simulink model "gm_parallel_8_phase_voltages"  (R2022a)
settings: Solver=FixedStepDiscrete  StartTime=0.0  StopTime=10.0  RelTol=1e-3
undefined symbols (not defined in the file or in its folder): f_c, u_dc
libraries: hdlmdlgenlib x14, simulink x2
(part 4 of 4)

== system gm_parallel_8_phase_voltages/Phase_voltages_per_switching_state1/Subsystem/MATLAB Function10/adder1 ==
  In1 : Inport
  In2 : Inport  Port=2
  adder1 : Sum  OutDataTypeStr=single  SampleTime=1e-08
  adder1_pd1 : Delay  DelayLength=6
  Out1 : Outport
  wires:
  In1/1 -> adder1/1
  In2/1 -> adder1/2
  adder1/1 -> adder1_pd1/1
  adder1_pd1/1 -> Out1/1

== system gm_parallel_8_phase_voltages/Phase_voltages_per_switching_state1/Subsystem/MATLAB Function10/adder2 ==
  In1 : Inport
  In2 : Inport  Port=2
  adder2 : Sum  OutDataTypeStr=single  SampleTime=1e-08
  adder2_pd1 : Delay  DelayLength=6
  Out1 : Outport
  wires:
  In1/1 -> adder2/1
  In2/1 -> adder2/2
  adder2/1 -> adder2_pd1/1
  adder2_pd1/1 -> Out1/1

== system gm_parallel_8_phase_voltages/Phase_voltages_per_switching_state1/Subsystem/MATLAB Function10/multiplier ==
  In1 : Inport
  In2 : Inport  Port=2
  multiplier : Product  Inputs=**  OutDataTypeStr=single  SampleTime=1e-08
  multiplier_pd1 : Delay  DelayLength=6
  Out1 : Outport
  wires:
  In1/1 -> multiplier/1
  In2/1 -> multiplier/2
  multiplier/1 -> multiplier_pd1/1
  multiplier_pd1/1 -> Out1/1

== system gm_parallel_8_phase_voltages/Phase_voltages_per_switching_state1/Subsystem/MATLAB Function10/multiplier1 ==
  In1 : Inport
  In2 : Inport  Port=2
  multiplier1 : Product  Inputs=**  OutDataTypeStr=single  SampleTime=1e-08
  multiplier1_pd1 : Delay  DelayLength=6
  Out1 : Outport
  wires:
  In1/1 -> multiplier1/1
  In2/1 -> multiplier1/2
  multiplier1/1 -> multiplier1_pd1/1
  multiplier1_pd1/1 -> Out1/1

== system gm_parallel_8_phase_voltages/Phase_voltages_per_switching_state1/Subsystem/MATLAB Function10/multiplier2 ==
  In1 : Inport
  In2 : Inport  Port=2
  multiplier2 : Product  Inputs=**  OutDataTypeStr=single  SampleTime=1e-08
  multiplier2_pd1 : Delay  DelayLength=6
  Out1 : Outport
  wires:
  In1/1 -> multiplier2/1
  In2/1 -> multiplier2/2
  multiplier2/1 -> multiplier2_pd1/1
  multiplier2_pd1/1 -> Out1/1

== system gm_parallel_8_phase_voltages/Phase_voltages_per_switching_state1/Subsystem/MATLAB Function10/multiplier3 ==
  In1 : Inport
  In2 : Inport  Port=2
  multiplier3 : Product  Inputs=**  OutDataTypeStr=single  SampleTime=1e-08
  multiplier3_pd1 : Delay  DelayLength=6
  Out1 : Outport
  wires:
  In1/1 -> multiplier3/1
  In2/1 -> multiplier3/2
  multiplier3/1 -> multiplier3_pd1/1
  multiplier3_pd1/1 -> Out1/1

== system gm_parallel_8_phase_voltages/Phase_voltages_per_switching_state1/Subsystem/MATLAB Function10/multiplier4 ==
  In1 : Inport
  In2 : Inport  Port=2
  multiplier4 : Product  Inputs=**  OutDataTypeStr=single  SampleTime=1e-08
  multiplier4_pd1 : Delay  DelayLength=6
  Out1 : Outport
  wires:
  In1/1 -> multiplier4/1
  In2/1 -> multiplier4/2
  multiplier4/1 -> multiplier4_pd1/1
  multiplier4_pd1/1 -> Out1/1

== system gm_parallel_8_phase_voltages/Phase_voltages_per_switching_state1/Subsystem/MATLAB Function10/uminus ==
  In1 : Inport
  uminus : UnaryMinus  SampleTime=1e-08
  Out1 : Outport
  wires:
  In1/1 -> uminus/1
  uminus/1 -> Out1/1

== system gm_parallel_8_phase_voltages/Phase_voltages_per_switching_state1/Subsystem/MATLAB Function11/adder1 ==
  In1 : Inport
  In2 : Inport  Port=2
  adder1 : Sum  OutDataTypeStr=single  SampleTime=1e-08
  adder1_pd1 : Delay  DelayLength=6
  Out1 : Outport
  wires:
  In1/1 -> adder1/1
  In2/1 -> adder1/2
  adder1/1 -> adder1_pd1/1
  adder1_pd1/1 -> Out1/1

== system gm_parallel_8_phase_voltages/Phase_voltages_per_switching_state1/Subsystem/MATLAB Function11/adder2 ==
  In1 : Inport
  In2 : Inport  Port=2
  adder2 : Sum  OutDataTypeStr=single  SampleTime=1e-08
  adder2_pd1 : Delay  DelayLength=6
  Out1 : Outport
  wires:
  In1/1 -> adder2/1
  In2/1 -> adder2/2
  adder2/1 -> adder2_pd1/1
  adder2_pd1/1 -> Out1/1

== system gm_parallel_8_phase_voltages/Phase_voltages_per_switching_state1/Subsystem/MATLAB Function11/multiplier ==
  In1 : Inport
  In2 : Inport  Port=2
  multiplier : Product  Inputs=**  OutDataTypeStr=single  SampleTime=1e-08
  multiplier_pd1 : Delay  DelayLength=6
  Out1 : Outport
  wires:
  In1/1 -> multiplier/1
  In2/1 -> multiplier/2
  multiplier/1 -> multiplier_pd1/1
  multiplier_pd1/1 -> Out1/1

== system gm_parallel_8_phase_voltages/Phase_voltages_per_switching_state1/Subsystem/MATLAB Function11/multiplier1 ==
  In1 : Inport
  In2 : Inport  Port=2
  multiplier1 : Product  Inputs=**  OutDataTypeStr=single  SampleTime=1e-08
  multiplier1_pd1 : Delay  DelayLength=6
  Out1 : Outport
  wires:
  In1/1 -> multiplier1/1
  In2/1 -> multiplier1/2
  multiplier1/1 -> multiplier1_pd1/1
  multiplier1_pd1/1 -> Out1/1

== system gm_parallel_8_phase_voltages/Phase_voltages_per_switching_state1/Subsystem/MATLAB Function11/multiplier2 ==
  In1 : Inport
  In2 : Inport  Port=2
  multiplier2 : Product  Inputs=**  OutDataTypeStr=single  SampleTime=1e-08
  multiplier2_pd1 : Delay  DelayLength=6
  Out1 : Outport
  wires:
  In1/1 -> multiplier2/1
  In2/1 -> multiplier2/2
  multiplier2/1 -> multiplier2_pd1/1
  multiplier2_pd1/1 -> Out1/1

== system gm_parallel_8_phase_voltages/Phase_voltages_per_switching_state1/Subsystem/MATLAB Function11/multiplier3 ==
  In1 : Inport
  In2 : Inport  Port=2
  multiplier3 : Product  Inputs=**  OutDataTypeStr=single  SampleTime=1e-08
  multiplier3_pd1 : Delay  DelayLength=6
  Out1 : Outport
  wires:
  In1/1 -> multiplier3/1
  In2/1 -> multiplier3/2
  multiplier3/1 -> multiplier3_pd1/1
  multiplier3_pd1/1 -> Out1/1

== system gm_parallel_8_phase_voltages/Phase_voltages_per_switching_state1/Subsystem/MATLAB Function11/multiplier4 ==
  In1 : Inport
  In2 : Inport  Port=2
  multiplier4 : Product  Inputs=**  OutDataTypeStr=single  SampleTime=1e-08
  multiplier4_pd1 : Delay  DelayLength=6
  Out1 : Outport
  wires:
  In1/1 -> multiplier4/1
  In2/1 -> multiplier4/2
  multiplier4/1 -> multiplier4_pd1/1
  multiplier4_pd1/1 -> Out1/1

== system gm_parallel_8_phase_voltages/Phase_voltages_per_switching_state1/Subsystem/MATLAB Function11/uminus ==
  In1 : Inport
  uminus : UnaryMinus  SampleTime=1e-08
  Out1 : Outport
  wires:
  In1/1 -> uminus/1
  uminus/1 -> Out1/1

== system gm_parallel_8_phase_voltages/Phase_voltages_per_switching_state1/Subsystem/MATLAB Function12/adder1 ==
  In1 : Inport
  In2 : Inport  Port=2
  adder1 : Sum  OutDataTypeStr=single  SampleTime=1e-08
  adder1_pd1 : Delay  DelayLength=6
  Out1 : Outport
  wires:
  In1/1 -> adder1/1
  In2/1 -> adder1/2
  adder1/1 -> adder1_pd1/1
  adder1_pd1/1 -> Out1/1

== system gm_parallel_8_phase_voltages/Phase_voltages_per_switching_state1/Subsystem/MATLAB Function12/adder2 ==
  In1 : Inport
  In2 : Inport  Port=2
  adder2 : Sum  OutDataTypeStr=single  SampleTime=1e-08
  adder2_pd1 : Delay  DelayLength=6
  Out1 : Outport
  wires:
  In1/1 -> adder2/1
  In2/1 -> adder2/2
  adder2/1 -> adder2_pd1/1
  adder2_pd1/1 -> Out1/1

== system gm_parallel_8_phase_voltages/Phase_voltages_per_switching_state1/Subsystem/MATLAB Function12/multiplier ==
  In1 : Inport
  In2 : Inport  Port=2
  multiplier : Product  Inputs=**  OutDataTypeStr=single  SampleTime=1e-08
  multiplier_pd1 : Delay  DelayLength=6
  Out1 : Outport
  wires:
  In1/1 -> multiplier/1
  In2/1 -> multiplier/2
  multiplier/1 -> multiplier_pd1/1
  multiplier_pd1/1 -> Out1/1

== system gm_parallel_8_phase_voltages/Phase_voltages_per_switching_state1/Subsystem/MATLAB Function12/multiplier1 ==
  In1 : Inport
  In2 : Inport  Port=2
  multiplier1 : Product  Inputs=**  OutDataTypeStr=single  SampleTime=1e-08
  multiplier1_pd1 : Delay  DelayLength=6
  Out1 : Outport
  wires:
  In1/1 -> multiplier1/1
  In2/1 -> multiplier1/2
  multiplier1/1 -> multiplier1_pd1/1
  multiplier1_pd1/1 -> Out1/1

== system gm_parallel_8_phase_voltages/Phase_voltages_per_switching_state1/Subsystem/MATLAB Function12/multiplier2 ==
  In1 : Inport
  In2 : Inport  Port=2
  multiplier2 : Product  Inputs=**  OutDataTypeStr=single  SampleTime=1e-08
  multiplier2_pd1 : Delay  DelayLength=6
  Out1 : Outport
  wires:
  In1/1 -> multiplier2/1
  In2/1 -> multiplier2/2
  multiplier2/1 -> multiplier2_pd1/1
  multiplier2_pd1/1 -> Out1/1

== system gm_parallel_8_phase_voltages/Phase_voltages_per_switching_state1/Subsystem/MATLAB Function12/multiplier3 ==
  In1 : Inport
  In2 : Inport  Port=2
  multiplier3 : Product  Inputs=**  OutDataTypeStr=single  SampleTime=1e-08
  multiplier3_pd1 : Delay  DelayLength=6
  Out1 : Outport
  wires:
  In1/1 -> multiplier3/1
  In2/1 -> multiplier3/2
  multiplier3/1 -> multiplier3_pd1/1
  multiplier3_pd1/1 -> Out1/1

== system gm_parallel_8_phase_voltages/Phase_voltages_per_switching_state1/Subsystem/MATLAB Function12/multiplier4 ==
  In1 : Inport
  In2 : Inport  Port=2
  multiplier4 : Product  Inputs=**  OutDataTypeStr=single  SampleTime=1e-08
  multiplier4_pd1 : Delay  DelayLength=6
  Out1 : Outport
  wires:
  In1/1 -> multiplier4/1
  In2/1 -> multiplier4/2
  multiplier4/1 -> multiplier4_pd1/1
  multiplier4_pd1/1 -> Out1/1

== system gm_parallel_8_phase_voltages/Phase_voltages_per_switching_state1/Subsystem/MATLAB Function12/uminus ==
  In1 : Inport
  uminus : UnaryMinus  SampleTime=1e-08
  Out1 : Outport
  wires:
  In1/1 -> uminus/1
  uminus/1 -> Out1/1

== system gm_parallel_8_phase_voltages/Phase_voltages_per_switching_state1/Subsystem/MATLAB Function13/adder1 ==
  In1 : Inport
  In2 : Inport  Port=2
  adder1 : Sum  OutDataTypeStr=single  SampleTime=1e-08
  adder1_pd1 : Delay  DelayLength=6
  Out1 : Outport
  wires:
  In1/1 -> adder1/1
  In2/1 -> adder1/2
  adder1/1 -> adder1_pd1/1
  adder1_pd1/1 -> Out1/1

== system gm_parallel_8_phase_voltages/Phase_voltages_per_switching_state1/Subsystem/MATLAB Function13/adder2 ==
  In1 : Inport
  In2 : Inport  Port=2
  adder2 : Sum  OutDataTypeStr=single  SampleTime=1e-08
  adder2_pd1 : Delay  DelayLength=6
  Out1 : Outport
  wires:
  In1/1 -> adder2/1
  In2/1 -> adder2/2
  adder2/1 -> adder2_pd1/1
  adder2_pd1/1 -> Out1/1

== system gm_parallel_8_phase_voltages/Phase_voltages_per_switching_state1/Subsystem/MATLAB Function13/multiplier ==
  In1 : Inport
  In2 : Inport  Port=2
  multiplier : Product  Inputs=**  OutDataTypeStr=single  SampleTime=1e-08
  multiplier_pd1 : Delay  DelayLength=6
  Out1 : Outport
  wires:
  In1/1 -> multiplier/1
  In2/1 -> multiplier/2
  multiplier/1 -> multiplier_pd1/1
  multiplier_pd1/1 -> Out1/1

== system gm_parallel_8_phase_voltages/Phase_voltages_per_switching_state1/Subsystem/MATLAB Function13/multiplier1 ==
  In1 : Inport
  In2 : Inport  Port=2
  multiplier1 : Product  Inputs=**  OutDataTypeStr=single  SampleTime=1e-08
  multiplier1_pd1 : Delay  DelayLength=6
  Out1 : Outport
  wires:
  In1/1 -> multiplier1/1
  In2/1 -> multiplier1/2
  multiplier1/1 -> multiplier1_pd1/1
  multiplier1_pd1/1 -> Out1/1

== system gm_parallel_8_phase_voltages/Phase_voltages_per_switching_state1/Subsystem/MATLAB Function13/multiplier2 ==
  In1 : Inport
  In2 : Inport  Port=2
  multiplier2 : Product  Inputs=**  OutDataTypeStr=single  SampleTime=1e-08
  multiplier2_pd1 : Delay  DelayLength=6
  Out1 : Outport
  wires:
  In1/1 -> multiplier2/1
  In2/1 -> multiplier2/2
  multiplier2/1 -> multiplier2_pd1/1
  multiplier2_pd1/1 -> Out1/1

== system gm_parallel_8_phase_voltages/Phase_voltages_per_switching_state1/Subsystem/MATLAB Function13/multiplier3 ==
  In1 : Inport
  In2 : Inport  Port=2
  multiplier3 : Product  Inputs=**  OutDataTypeStr=single  SampleTime=1e-08
  multiplier3_pd1 : Delay  DelayLength=6
  Out1 : Outport
  wires:
  In1/1 -> multiplier3/1
  In2/1 -> multiplier3/2
  multiplier3/1 -> multiplier3_pd1/1
  multiplier3_pd1/1 -> Out1/1

== system gm_parallel_8_phase_voltages/Phase_voltages_per_switching_state1/Subsystem/MATLAB Function13/multiplier4 ==
  In1 : Inport
  In2 : Inport  Port=2
  multiplier4 : Product  Inputs=**  OutDataTypeStr=single  SampleTime=1e-08
  multiplier4_pd1 : Delay  DelayLength=6
  Out1 : Outport
  wires:
  In1/1 -> multiplier4/1
  In2/1 -> multiplier4/2
  multiplier4/1 -> multiplier4_pd1/1
  multiplier4_pd1/1 -> Out1/1

== system gm_parallel_8_phase_voltages/Phase_voltages_per_switching_state1/Subsystem/MATLAB Function13/uminus ==
  In1 : Inport
  uminus : UnaryMinus  SampleTime=1e-08
  Out1 : Outport
  wires:
  In1/1 -> uminus/1
  uminus/1 -> Out1/1

== system gm_parallel_8_phase_voltages/Phase_voltages_per_switching_state1/Subsystem/MATLAB Function14/adder1 ==
  In1 : Inport
  In2 : Inport  Port=2
  adder1 : Sum  OutDataTypeStr=single  SampleTime=1e-08
  adder1_pd1 : Delay  DelayLength=6
  Out1 : Outport
  wires:
  In1/1 -> adder1/1
  In2/1 -> adder1/2
  adder1/1 -> adder1_pd1/1
  adder1_pd1/1 -> Out1/1

== system gm_parallel_8_phase_voltages/Phase_voltages_per_switching_state1/Subsystem/MATLAB Function14/adder2 ==
  In1 : Inport
  In2 : Inport  Port=2
  adder2 : Sum  OutDataTypeStr=single  SampleTime=1e-08
  adder2_pd1 : Delay  DelayLength=6
  Out1 : Outport
  wires:
  In1/1 -> adder2/1
  In2/1 -> adder2/2
  adder2/1 -> adder2_pd1/1
  adder2_pd1/1 -> Out1/1

== system gm_parallel_8_phase_voltages/Phase_voltages_per_switching_state1/Subsystem/MATLAB Function14/multiplier ==
  In1 : Inport
  In2 : Inport  Port=2
  multiplier : Product  Inputs=**  OutDataTypeStr=single  SampleTime=1e-08
  multiplier_pd1 : Delay  DelayLength=6
  Out1 : Outport
  wires:
  In1/1 -> multiplier/1
  In2/1 -> multiplier/2
  multiplier/1 -> multiplier_pd1/1
  multiplier_pd1/1 -> Out1/1

== system gm_parallel_8_phase_voltages/Phase_voltages_per_switching_state1/Subsystem/MATLAB Function14/multiplier1 ==
  In1 : Inport
  In2 : Inport  Port=2
  multiplier1 : Product  Inputs=**  OutDataTypeStr=single  SampleTime=1e-08
  multiplier1_pd1 : Delay  DelayLength=6
  Out1 : Outport
  wires:
  In1/1 -> multiplier1/1
  In2/1 -> multiplier1/2
  multiplier1/1 -> multiplier1_pd1/1
  multiplier1_pd1/1 -> Out1/1

== system gm_parallel_8_phase_voltages/Phase_voltages_per_switching_state1/Subsystem/MATLAB Function14/multiplier2 ==
  In1 : Inport
  In2 : Inport  Port=2
  multiplier2 : Product  Inputs=**  OutDataTypeStr=single  SampleTime=1e-08
  multiplier2_pd1 : Delay  DelayLength=6
  Out1 : Outport
  wires:
  In1/1 -> multiplier2/1
  In2/1 -> multiplier2/2
  multiplier2/1 -> multiplier2_pd1/1
  multiplier2_pd1/1 -> Out1/1

== system gm_parallel_8_phase_voltages/Phase_voltages_per_switching_state1/Subsystem/MATLAB Function14/multiplier3 ==
  In1 : Inport
  In2 : Inport  Port=2
  multiplier3 : Product  Inputs=**  OutDataTypeStr=single  SampleTime=1e-08
  multiplier3_pd1 : Delay  DelayLength=6
  Out1 : Outport
  wires:
  In1/1 -> multiplier3/1
  In2/1 -> multiplier3/2
  multiplier3/1 -> multiplier3_pd1/1
  multiplier3_pd1/1 -> Out1/1

== system gm_parallel_8_phase_voltages/Phase_voltages_per_switching_state1/Subsystem/MATLAB Function14/multiplier4 ==
  In1 : Inport
  In2 : Inport  Port=2
  multiplier4 : Product  Inputs=**  OutDataTypeStr=single  SampleTime=1e-08
  multiplier4_pd1 : Delay  DelayLength=6
  Out1 : Outport
  wires:
  In1/1 -> multiplier4/1
  In2/1 -> multiplier4/2
  multiplier4/1 -> multiplier4_pd1/1
  multiplier4_pd1/1 -> Out1/1

== system gm_parallel_8_phase_voltages/Phase_voltages_per_switching_state1/Subsystem/MATLAB Function14/uminus ==
  In1 : Inport
  uminus : UnaryMinus  SampleTime=1e-08
  Out1 : Outport
  wires:
  In1/1 -> uminus/1
  uminus/1 -> Out1/1

== system gm_parallel_8_phase_voltages/Phase_voltages_per_switching_state1/Subsystem/MATLAB Function15/adder1 ==
  In1 : Inport
  In2 : Inport  Port=2
  adder1 : Sum  OutDataTypeStr=single  SampleTime=1e-08
  adder1_pd1 : Delay  DelayLength=6
  Out1 : Outport
  wires:
  In1/1 -> adder1/1
  In2/1 -> adder1/2
  adder1/1 -> adder1_pd1/1
  adder1_pd1/1 -> Out1/1

== system gm_parallel_8_phase_voltages/Phase_voltages_per_switching_state1/Subsystem/MATLAB Function15/adder2 ==
  In1 : Inport
  In2 : Inport  Port=2
  adder2 : Sum  OutDataTypeStr=single  SampleTime=1e-08
  adder2_pd1 : Delay  DelayLength=6
  Out1 : Outport
  wires:
  In1/1 -> adder2/1
  In2/1 -> adder2/2
  adder2/1 -> adder2_pd1/1
  adder2_pd1/1 -> Out1/1

== system gm_parallel_8_phase_voltages/Phase_voltages_per_switching_state1/Subsystem/MATLAB Function15/multiplier ==
  In1 : Inport
  In2 : Inport  Port=2
  multiplier : Product  Inputs=**  OutDataTypeStr=single  SampleTime=1e-08
  multiplier_pd1 : Delay  DelayLength=6
  Out1 : Outport
  wires:
  In1/1 -> multiplier/1
  In2/1 -> multiplier/2
  multiplier/1 -> multiplier_pd1/1
  multiplier_pd1/1 -> Out1/1

== system gm_parallel_8_phase_voltages/Phase_voltages_per_switching_state1/Subsystem/MATLAB Function15/multiplier1 ==
  In1 : Inport
  In2 : Inport  Port=2
  multiplier1 : Product  Inputs=**  OutDataTypeStr=single  SampleTime=1e-08
  multiplier1_pd1 : Delay  DelayLength=6
  Out1 : Outport
  wires:
  In1/1 -> multiplier1/1
  In2/1 -> multiplier1/2
  multiplier1/1 -> multiplier1_pd1/1
  multiplier1_pd1/1 -> Out1/1

== system gm_parallel_8_phase_voltages/Phase_voltages_per_switching_state1/Subsystem/MATLAB Function15/multiplier2 ==
  In1 : Inport
  In2 : Inport  Port=2
  multiplier2 : Product  Inputs=**  OutDataTypeStr=single  SampleTime=1e-08
  multiplier2_pd1 : Delay  DelayLength=6
  Out1 : Outport
  wires:
  In1/1 -> multiplier2/1
  In2/1 -> multiplier2/2
  multiplier2/1 -> multiplier2_pd1/1
  multiplier2_pd1/1 -> Out1/1

== system gm_parallel_8_phase_voltages/Phase_voltages_per_switching_state1/Subsystem/MATLAB Function15/multiplier3 ==
  In1 : Inport
  In2 : Inport  Port=2
  multiplier3 : Product  Inputs=**  OutDataTypeStr=single  SampleTime=1e-08
  multiplier3_pd1 : Delay  DelayLength=6
  Out1 : Outport
  wires:
  In1/1 -> multiplier3/1
  In2/1 -> multiplier3/2
  multiplier3/1 -> multiplier3_pd1/1
  multiplier3_pd1/1 -> Out1/1

== system gm_parallel_8_phase_voltages/Phase_voltages_per_switching_state1/Subsystem/MATLAB Function15/multiplier4 ==
  In1 : Inport
  In2 : Inport  Port=2
  multiplier4 : Product  Inputs=**  OutDataTypeStr=single  SampleTime=1e-08
  multiplier4_pd1 : Delay  DelayLength=6
  Out1 : Outport
  wires:
  In1/1 -> multiplier4/1
  In2/1 -> multiplier4/2
  multiplier4/1 -> multiplier4_pd1/1
  multiplier4_pd1/1 -> Out1/1

== system gm_parallel_8_phase_voltages/Phase_voltages_per_switching_state1/Subsystem/MATLAB Function15/uminus ==
  In1 : Inport
  uminus : UnaryMinus  SampleTime=1e-08
  Out1 : Outport
  wires:
  In1/1 -> uminus/1
  uminus/1 -> Out1/1

== system gm_parallel_8_phase_voltages/Phase_voltages_per_switching_state1/Subsystem/MATLAB Function8/adder1 ==
  In1 : Inport
  In2 : Inport  Port=2
  adder1 : Sum  OutDataTypeStr=single  SampleTime=1e-08
  adder1_pd1 : Delay  DelayLength=6
  Out1 : Outport
  wires:
  In1/1 -> adder1/1
  In2/1 -> adder1/2
  adder1/1 -> adder1_pd1/1
  adder1_pd1/1 -> Out1/1

== system gm_parallel_8_phase_voltages/Phase_voltages_per_switching_state1/Subsystem/MATLAB Function8/adder2 ==
  In1 : Inport
  In2 : Inport  Port=2
  adder2 : Sum  OutDataTypeStr=single  SampleTime=1e-08
  adder2_pd1 : Delay  DelayLength=6
  Out1 : Outport
  wires:
  In1/1 -> adder2/1
  In2/1 -> adder2/2
  adder2/1 -> adder2_pd1/1
  adder2_pd1/1 -> Out1/1

== system gm_parallel_8_phase_voltages/Phase_voltages_per_switching_state1/Subsystem/MATLAB Function8/multiplier ==
  In1 : Inport
  In2 : Inport  Port=2
  multiplier : Product  Inputs=**  OutDataTypeStr=single  SampleTime=1e-08
  multiplier_pd1 : Delay  DelayLength=6
  Out1 : Outport
  wires:
  In1/1 -> multiplier/1
  In2/1 -> multiplier/2
  multiplier/1 -> multiplier_pd1/1
  multiplier_pd1/1 -> Out1/1

== system gm_parallel_8_phase_voltages/Phase_voltages_per_switching_state1/Subsystem/MATLAB Function8/multiplier1 ==
  In1 : Inport
  In2 : Inport  Port=2
  multiplier1 : Product  Inputs=**  OutDataTypeStr=single  SampleTime=1e-08
  multiplier1_pd1 : Delay  DelayLength=6
  Out1 : Outport
  wires:
  In1/1 -> multiplier1/1
  In2/1 -> multiplier1/2
  multiplier1/1 -> multiplier1_pd1/1
  multiplier1_pd1/1 -> Out1/1

== system gm_parallel_8_phase_voltages/Phase_voltages_per_switching_state1/Subsystem/MATLAB Function8/multiplier2 ==
  In1 : Inport
  In2 : Inport  Port=2
  multiplier2 : Product  Inputs=**  OutDataTypeStr=single  SampleTime=1e-08
  multiplier2_pd1 : Delay  DelayLength=6
  Out1 : Outport
  wires:
  In1/1 -> multiplier2/1
  In2/1 -> multiplier2/2
  multiplier2/1 -> multiplier2_pd1/1
  multiplier2_pd1/1 -> Out1/1

== system gm_parallel_8_phase_voltages/Phase_voltages_per_switching_state1/Subsystem/MATLAB Function8/multiplier3 ==
  In1 : Inport
  In2 : Inport  Port=2
  multiplier3 : Product  Inputs=**  OutDataTypeStr=single  SampleTime=1e-08
  multiplier3_pd1 : Delay  DelayLength=6
  Out1 : Outport
  wires:
  In1/1 -> multiplier3/1
  In2/1 -> multiplier3/2
  multiplier3/1 -> multiplier3_pd1/1
  multiplier3_pd1/1 -> Out1/1

== system gm_parallel_8_phase_voltages/Phase_voltages_per_switching_state1/Subsystem/MATLAB Function8/multiplier4 ==
  In1 : Inport
  In2 : Inport  Port=2
  multiplier4 : Product  Inputs=**  OutDataTypeStr=single  SampleTime=1e-08
  multiplier4_pd1 : Delay  DelayLength=6
  Out1 : Outport
  wires:
  In1/1 -> multiplier4/1
  In2/1 -> multiplier4/2
  multiplier4/1 -> multiplier4_pd1/1
  multiplier4_pd1/1 -> Out1/1

== system gm_parallel_8_phase_voltages/Phase_voltages_per_switching_state1/Subsystem/MATLAB Function8/uminus ==
  In1 : Inport
  uminus : UnaryMinus  SampleTime=1e-08
  Out1 : Outport
  wires:
  In1/1 -> uminus/1
  uminus/1 -> Out1/1

== system gm_parallel_8_phase_voltages/Phase_voltages_per_switching_state1/Subsystem/MATLAB Function9/adder1 ==
  In1 : Inport
  In2 : Inport  Port=2
  adder1 : Sum  OutDataTypeStr=single  SampleTime=1e-08
  adder1_pd1 : Delay  DelayLength=6
  Out1 : Outport
  wires:
  In1/1 -> adder1/1
  In2/1 -> adder1/2
  adder1/1 -> adder1_pd1/1
  adder1_pd1/1 -> Out1/1

== system gm_parallel_8_phase_voltages/Phase_voltages_per_switching_state1/Subsystem/MATLAB Function9/adder2 ==
  In1 : Inport
  In2 : Inport  Port=2
  adder2 : Sum  OutDataTypeStr=single  SampleTime=1e-08
  adder2_pd1 : Delay  DelayLength=6
  Out1 : Outport
  wires:
  In1/1 -> adder2/1
  In2/1 -> adder2/2
  adder2/1 -> adder2_pd1/1
  adder2_pd1/1 -> Out1/1

== system gm_parallel_8_phase_voltages/Phase_voltages_per_switching_state1/Subsystem/MATLAB Function9/multiplier ==
  In1 : Inport
  In2 : Inport  Port=2
  multiplier : Product  Inputs=**  OutDataTypeStr=single  SampleTime=1e-08
  multiplier_pd1 : Delay  DelayLength=6
  Out1 : Outport
  wires:
  In1/1 -> multiplier/1
  In2/1 -> multiplier/2
  multiplier/1 -> multiplier_pd1/1
  multiplier_pd1/1 -> Out1/1

== system gm_parallel_8_phase_voltages/Phase_voltages_per_switching_state1/Subsystem/MATLAB Function9/multiplier1 ==
  In1 : Inport
  In2 : Inport  Port=2
  multiplier1 : Product  Inputs=**  OutDataTypeStr=single  SampleTime=1e-08
  multiplier1_pd1 : Delay  DelayLength=6
  Out1 : Outport
  wires:
  In1/1 -> multiplier1/1
  In2/1 -> multiplier1/2
  multiplier1/1 -> multiplier1_pd1/1
  multiplier1_pd1/1 -> Out1/1

== system gm_parallel_8_phase_voltages/Phase_voltages_per_switching_state1/Subsystem/MATLAB Function9/multiplier2 ==
  In1 : Inport
  In2 : Inport  Port=2
  multiplier2 : Product  Inputs=**  OutDataTypeStr=single  SampleTime=1e-08
  multiplier2_pd1 : Delay  DelayLength=6
  Out1 : Outport
  wires:
  In1/1 -> multiplier2/1
  In2/1 -> multiplier2/2
  multiplier2/1 -> multiplier2_pd1/1
  multiplier2_pd1/1 -> Out1/1

== system gm_parallel_8_phase_voltages/Phase_voltages_per_switching_state1/Subsystem/MATLAB Function9/multiplier3 ==
  In1 : Inport
  In2 : Inport  Port=2
  multiplier3 : Product  Inputs=**  OutDataTypeStr=single  SampleTime=1e-08
  multiplier3_pd1 : Delay  DelayLength=6
  Out1 : Outport
  wires:
  In1/1 -> multiplier3/1
  In2/1 -> multiplier3/2
  multiplier3/1 -> multiplier3_pd1/1
  multiplier3_pd1/1 -> Out1/1

== system gm_parallel_8_phase_voltages/Phase_voltages_per_switching_state1/Subsystem/MATLAB Function9/multiplier4 ==
  In1 : Inport
  In2 : Inport  Port=2
  multiplier4 : Product  Inputs=**  OutDataTypeStr=single  SampleTime=1e-08
  multiplier4_pd1 : Delay  DelayLength=6
  Out1 : Outport
  wires:
  In1/1 -> multiplier4/1
  In2/1 -> multiplier4/2
  multiplier4/1 -> multiplier4_pd1/1
  multiplier4_pd1/1 -> Out1/1

== system gm_parallel_8_phase_voltages/Phase_voltages_per_switching_state1/Subsystem/MATLAB Function9/uminus ==
  In1 : Inport
  uminus : UnaryMinus  SampleTime=1e-08
  Out1 : Outport
  wires:
  In1/1 -> uminus/1
  uminus/1 -> Out1/1
